simulink model "galvoMdl2"  (R2013a)
settings: Solver=ode45  StartTime=0.0  StopTime=10.0  RelTol=1e-3
undefined symbols (not defined in the file): BF, JR, KME, L, RL
settings Model: Creator=mainster  LastModifiedBy=mainster

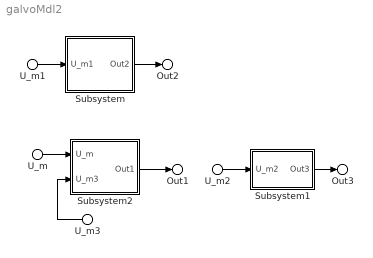
== system galvoMdl2 ==
  U_m : Inport
  U_m2 : Inport  Port=2
  U_m3 : Inport  Port=3
  U_m1 : Inport  Port=4
  Subsystem : Subsystem
  Subsystem1 : Subsystem
  Subsystem2 : Subsystem
  Out1 : Outport
  Out3 : Outport  Port=2
  Out2 : Outport  Port=3
  wires:
  U_m1/1 -> Subsystem/1(U_m1)
  Subsystem/1(Out2) -> Out2/1
  U_m2/1 -> Subsystem1/1(U_m2)
  Subsystem1/1(Out3) -> Out3/1
  U_m/1 -> Subsystem2/1(U_m)
  U_m3/1 -> Subsystem2/2(U_m3)
  Subsystem2/1(Out1) -> Out1/1

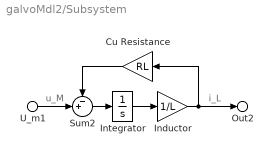
== system galvoMdl2/Subsystem ==
  note: u_M
  note: i_L
  U_m1 : Inport
  Cu Resistance : Gain  Gain=RL
  Inductor : Gain  Gain=1/L
  Integrator : Integrator
  Sum2 : Sum  Inputs=-+|
  Out2 : Outport
  wires:
  U_m1/1 -> Sum2/2
  Sum2/1 -> Integrator/1
  Inductor/1 -> Out2/1, Cu Resistance/1
  Integrator/1 -> Inductor/1
  Cu Resistance/1 -> Sum2/1

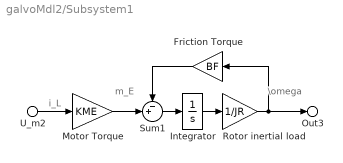
== system galvoMdl2/Subsystem1 ==
  note: m_E
  note: \omega
  note: i_L
  U_m2 : Inport
  Friction Torque : Gain  Gain=BF
  Integrator : Integrator
  Motor Torque : Gain  Gain=KME
  Rotor inertial load : Gain  Gain=1/JR
  Sum1 : Sum  Inputs=-+|
  Out3 : Outport
  wires:
  Sum1/1 -> Integrator/1
  Integrator/1 -> Rotor inertial load/1
  Friction Torque/1 -> Sum1/1
  U_m2/1 -> Motor Torque/1
  Motor Torque/1 -> Sum1/2
  Rotor inertial load/1 -> Out3/1, Friction Torque/1

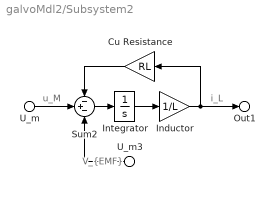
== system galvoMdl2/Subsystem2 ==
  note: u_M
  note: i_L
  note: V_{EMF}
  U_m : Inport
  U_m3 : Inport  Port=2
  Cu Resistance : Gain  Gain=RL
  Inductor : Gain  Gain=1/L
  Integrator : Integrator
  Sum2 : Sum  Inputs=-+-
  Out1 : Outport
  wires:
  Sum2/1 -> Integrator/1
  Cu Resistance/1 -> Sum2/1
  Integrator/1 -> Inductor/1
  U_m3/1 -> Sum2/3
  U_m/1 -> Sum2/2
  Inductor/1 -> Out1/1, Cu Resistance/1
